simulink model "distributive4"  (R2022b)
settings: Solver=ode8  StartTime=0.0  StopTime=0.25  FixedStep=0.0001  RelTol=1e-3
values from neighbouring files (symbols this model uses):
  A = [a11,0;0,a22]    [distributive3.m]    (also in neurobserver4.m = [1 1;1 2])
  alpha = 0.9e-6    (= 9e-07)    [distributive3.m]
  amp = 80e-6    (= 8e-05)    [distributive3.m]
  angvel = (2*pi)*30    (= 188.495559215)    [distributive3.m]
  B = [b11,0;0,b22]    [distributive3.m]    (also in neurobserver4.m = 1000)
  beta = 0.008    [distributive3.m]
  C = [1,0]    [distributive3.m]
  C_bar = [1,0]    [distributive3.m]    (also in neurobserver4.m = [1,0;0,1])
  d_p = 1.6e-6    (= 1.6e-06)    [distributive3.m]
  fase = 2*pi/10    (= 0.628318530718)    [distributive3.m]
  G = S\C_bar'    [distributive3.m]    (also in neurobserver4.m)
  gamma = 0.008    [distributive3.m]
  Gamma = [0,-B;0 0]    [distributive3.m]    (also in neurobserver4.m = [ 0 , -B ; 0 , 0 ])
  h = legend('Closed-loop response map $(y_d,y)$')    [distributive3.m]    (also in neurobserver4.m = legend('$(y_r,y)$ for $x=7.5$, $f=1Hz$','$(y_r,y)$ for $x=15)
  h_i = 2e-6    (= 2e-06)    [distributive3.m]
  k1 = 7    [distributive3.m]    (also in neurobserver4.m)
  k2 = 7    [distributive3.m]    (also in neurobserver4.m)
  kappa1 = 4e3    (= 4000)    [distributive3.m]    (also in neurobserver4.m = 120)
  L = 20000    [distributive3.m]
  S = [s11,s12;s21,s22]    [distributive3.m]    (also in neurobserver4.m = [1/theta,B/theta^2;B/theta^2,(2*B^2)/theta^3])
  V = learning.V    [neurobserver4.m]
  W = learning.W    [neurobserver4.m]
  x1 = e(2)    [distributive3.m]
  x2 = e(5)    [distributive3.m]
  y_i = -3e-6    (= -3e-06)    [distributive3.m]
undefined symbols (not defined in the file or in its folder): freq, Gamma_c, Y
(part 2 of 3)

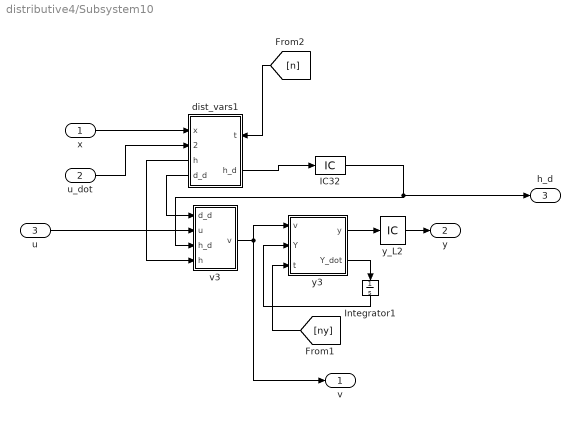
== system distributive4/Subsystem10 ==
  x : Inport
  u_dot : Inport  Port=2
  u : Inport  Port=3
  IC32 : InitialCondition  Value=h_i
  Integrator1 : Integrator
  dist_vars1 : Subsystem
      settings: PortSchema="{\"entries\":[{\"content\":{\"sides\":[{\"content\":{\"connectorIds\":[\"In1\",\"In2\",\"Out2\",\"Out3\"]},\"type\":\"ConnectorPlacement.EquallySpacedRectSide\",\"uuid\":\"c6804a03-85ed-4e19-a8b2-23b3b91cc999\"},{\"content\":{\"connectorIds\":[\"In3\",\"Out1\"],\"side\":\"RIGHT\"},\"type\":\"ConnectorPlacement.EquallySpacedRectSide\",\"uuid\":\"3893e005-dabd-44b9-aa2f-690b9b6a2b6d\"},{\"content\":{\"connectorIds\":[],\"side\":\"TOP\"},\"type\":\"ConnectorPlacement.EquallySpacedRectSide\",\"uuid\":\"9986ad97-c002-4a16-bb79-a95333cc5799\"}]},\"type\":\"ConnectorPlacement.EquallySpacedConnector\",\"uuid\":\"d796f436-4cc2-4114-998c-ef0d57f68d4d\"}],\"packageUris\":[\"http://schema.mathworks.com/mf0/Connector/R2020b\"],\"version\":\"1.0\"}"
  v3 : MATLAB Function  TreatAsAtomicUnit=on
  y3 : MATLAB Function  TreatAsAtomicUnit=on
  y_L2 : InitialCondition  Value=[y_i;0]
  v : Outport
  y : Outport  Port=2
  h_d : Outport  Port=3
  wires:
  dist_vars1/3(d_d) -> v3/1(d_d)
  v3/1(v) -> y3/1(v), v/1
  y3/2(Y_dot) -> Integrator1/1
  IC32/1 -> v3/3(h_d), h_d/1
  dist_vars1/2(h) -> v3/4(h)
  dist_vars1/1(h_d) -> IC32/1
  y3/1(y) -> y_L2/1
  [n] -> dist_vars1/3(t)
  Integrator1/1 -> y3/2(Y)
  [ny] -> y3/3(t)
  u_dot/1 -> dist_vars1/2(u_dot)
  x/1 -> dist_vars1/1(x)
  u/1 -> v3/2(u)
  y_L2/1 -> y/1

== system distributive4/Subsystem11 ==
  x : Inport
  y_ref : Inport  Port=2
  z_hat : Inport  Port=3
  d_d : Inport  Port=4
  Derivative32 : Derivative
  h_d_ref14 : MATLAB Function  TreatAsAtomicUnit=on
  u_ref13 : Integrator
  u_ref_dot14 : MATLAB Function  TreatAsAtomicUnit=on
  u_ref_dot : Outport
  u_ref : Outport  Port=2
  h_d_ref : Outport  Port=3
  wires:
  z_hat/1 -> h_d_ref14/4(z_hat), u_ref_dot14/2(z_hat)
  u_ref13/1 -> u_ref/1, h_d_ref14/1(u)
  Derivative32/1 -> h_d_ref14/3(y_ref_dot)
  x/1 -> u_ref_dot14/3(x)
  h_d_ref14/1(h_d_ref) -> u_ref_dot14/1(h_d_ref), h_d_ref/1
  u_ref_dot14/1(u_ref_dot) -> u_ref13/1, u_ref_dot/1
  d_d/1 -> h_d_ref14/5(d_d)
  y_ref/1 -> Derivative32/1, h_d_ref14/2(y_ref)

== system distributive4/Subsystem12 ==
  x : Inport
  y : Inport  Port=2
  u_dot : Inport  Port=3
  u : Inport  Port=4
  Integrator14 : Integrator  InitialCondition=[0;0]
  dist_vars15 : Subsystem
      settings: PortSchema="{\"entries\":[{\"content\":{\"sides\":[{\"content\":{\"connectorIds\":[\"In1\",\"In2\",\"Out1\",\"Out2\",\"Out3\"]},\"type\":\"ConnectorPlacement.EquallySpacedRectSide\",\"uuid\":\"c6804a03-85ed-4e19-a8b2-23b3b91cc999\"},{\"content\":{\"connectorIds\":[],\"side\":\"RIGHT\"},\"type\":\"ConnectorPlacement.EquallySpacedRectSide\",\"uuid\":\"3893e005-dabd-44b9-aa2f-690b9b6a2b6d\"},{\"content\":{\"connectorIds\":[],\"side\":\"TOP\"},\"type\":\"ConnectorPlacement.EquallySpacedRectSide\",\"uuid\":\"9986ad97-c002-4a16-bb79-a95333cc5799\"}]},\"type\":\"ConnectorPlacement.EquallySpacedConnector\",\"uuid\":\"d796f436-4cc2-4114-998c-ef0d57f68d4d\"}],\"packageUris\":[\"http://schema.mathworks.com/mf0/Connector/R2020b\"],\"version\":\"1.0\"}"
  observer5 : MATLAB Function  TreatAsAtomicUnit=on
  d_d : Outport
  z_hat : Outport  Port=2
  wires:
  observer5/1(z_hat_dot) -> Integrator14/1
  u/1 -> observer5/5(u)
  dist_vars15/3(h_d) -> observer5/4(h_d)
  dist_vars15/2(d_d) -> observer5/7(d_d), d_d/1
  dist_vars15/1(h_d_dot) -> observer5/6(h_d_dot)
  Integrator14/1 -> observer5/1(z_hat), z_hat/1
  u_dot/1 -> dist_vars15/1(u_dot)
  y/1 -> observer5/2(y)
  x/1 -> dist_vars15/2(x), observer5/3(x)

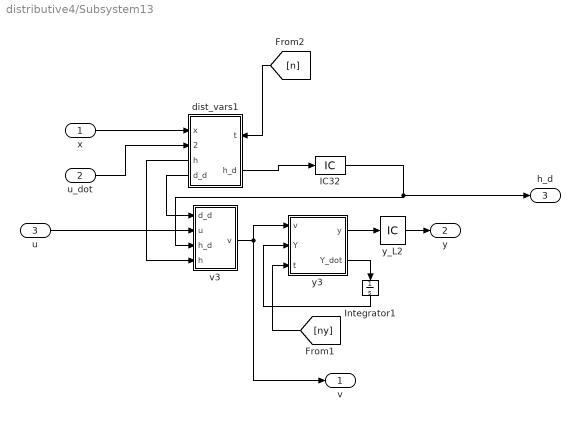
== system distributive4/Subsystem13 ==
  x : Inport
  u_dot : Inport  Port=2
  u : Inport  Port=3
  IC32 : InitialCondition  Value=h_i
  Integrator1 : Integrator
  dist_vars1 : Subsystem
      settings: PortSchema="{\"entries\":[{\"content\":{\"sides\":[{\"content\":{\"connectorIds\":[\"In1\",\"In2\",\"Out2\",\"Out3\"]},\"type\":\"ConnectorPlacement.EquallySpacedRectSide\",\"uuid\":\"c6804a03-85ed-4e19-a8b2-23b3b91cc999\"},{\"content\":{\"connectorIds\":[\"In3\",\"Out1\"],\"side\":\"RIGHT\"},\"type\":\"ConnectorPlacement.EquallySpacedRectSide\",\"uuid\":\"3893e005-dabd-44b9-aa2f-690b9b6a2b6d\"},{\"content\":{\"connectorIds\":[],\"side\":\"TOP\"},\"type\":\"ConnectorPlacement.EquallySpacedRectSide\",\"uuid\":\"9986ad97-c002-4a16-bb79-a95333cc5799\"}]},\"type\":\"ConnectorPlacement.EquallySpacedConnector\",\"uuid\":\"d796f436-4cc2-4114-998c-ef0d57f68d4d\"}],\"packageUris\":[\"http://schema.mathworks.com/mf0/Connector/R2020b\"],\"version\":\"1.0\"}"
  v3 : MATLAB Function  TreatAsAtomicUnit=on
  y3 : MATLAB Function  TreatAsAtomicUnit=on
  y_L2 : InitialCondition  Value=[y_i;0]
  v : Outport
  y : Outport  Port=2
  h_d : Outport  Port=3
  wires:
  dist_vars1/3(d_d) -> v3/1(d_d)
  v3/1(v) -> y3/1(v), v/1
  y3/2(Y_dot) -> Integrator1/1
  IC32/1 -> v3/3(h_d), h_d/1
  dist_vars1/2(h) -> v3/4(h)
  dist_vars1/1(h_d) -> IC32/1
  y3/1(y) -> y_L2/1
  [n] -> dist_vars1/3(t)
  Integrator1/1 -> y3/2(Y)
  [ny] -> y3/3(t)
  u_dot/1 -> dist_vars1/2(u_dot)
  x/1 -> dist_vars1/1(x)
  u/1 -> v3/2(u)
  y_L2/1 -> y/1

== system distributive4/Subsystem14 ==
  x : Inport
  y_ref : Inport  Port=2
  z_hat : Inport  Port=3
  d_d : Inport  Port=4
  Derivative32 : Derivative
  h_d_ref14 : MATLAB Function  TreatAsAtomicUnit=on
  u_ref13 : Integrator
  u_ref_dot14 : MATLAB Function  TreatAsAtomicUnit=on
  u_ref_dot : Outport
  u_ref : Outport  Port=2
  h_d_ref : Outport  Port=3
  wires:
  z_hat/1 -> h_d_ref14/4(z_hat), u_ref_dot14/2(z_hat)
  u_ref13/1 -> u_ref/1, h_d_ref14/1(u)
  Derivative32/1 -> h_d_ref14/3(y_ref_dot)
  x/1 -> u_ref_dot14/3(x)
  h_d_ref14/1(h_d_ref) -> u_ref_dot14/1(h_d_ref), h_d_ref/1
  u_ref_dot14/1(u_ref_dot) -> u_ref13/1, u_ref_dot/1
  d_d/1 -> h_d_ref14/5(d_d)
  y_ref/1 -> Derivative32/1, h_d_ref14/2(y_ref)

== system distributive4/Subsystem15 ==
  x : Inport
  y : Inport  Port=2
  u_dot : Inport  Port=3
  u : Inport  Port=4
  Integrator14 : Integrator  InitialCondition=[0;0]
  dist_vars15 : Subsystem
      settings: PortSchema="{\"entries\":[{\"content\":{\"sides\":[{\"content\":{\"connectorIds\":[\"In1\",\"In2\",\"Out1\",\"Out2\",\"Out3\"]},\"type\":\"ConnectorPlacement.EquallySpacedRectSide\",\"uuid\":\"c6804a03-85ed-4e19-a8b2-23b3b91cc999\"},{\"content\":{\"connectorIds\":[],\"side\":\"RIGHT\"},\"type\":\"ConnectorPlacement.EquallySpacedRectSide\",\"uuid\":\"3893e005-dabd-44b9-aa2f-690b9b6a2b6d\"},{\"content\":{\"connectorIds\":[],\"side\":\"TOP\"},\"type\":\"ConnectorPlacement.EquallySpacedRectSide\",\"uuid\":\"9986ad97-c002-4a16-bb79-a95333cc5799\"}]},\"type\":\"ConnectorPlacement.EquallySpacedConnector\",\"uuid\":\"d796f436-4cc2-4114-998c-ef0d57f68d4d\"}],\"packageUris\":[\"http://schema.mathworks.com/mf0/Connector/R2020b\"],\"version\":\"1.0\"}"
  observer5 : MATLAB Function  TreatAsAtomicUnit=on
  d_d : Outport
  z_hat : Outport  Port=2
  wires:
  observer5/1(z_hat_dot) -> Integrator14/1
  u/1 -> observer5/5(u)
  dist_vars15/3(h_d) -> observer5/4(h_d)
  dist_vars15/2(d_d) -> observer5/7(d_d), d_d/1
  dist_vars15/1(h_d_dot) -> observer5/6(h_d_dot)
  Integrator14/1 -> observer5/1(z_hat), z_hat/1
  u_dot/1 -> dist_vars15/1(u_dot)
  y/1 -> observer5/2(y)
  x/1 -> dist_vars15/2(x), observer5/3(x)

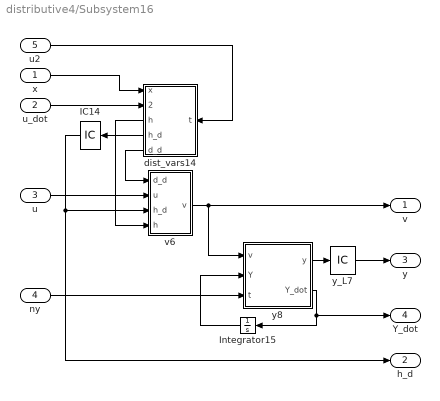
== system distributive4/Subsystem16 ==
  x : Inport
  u_dot : Inport  Port=2
  u : Inport  Port=3
  ny : Inport  Port=4
  u2 : Inport  Port=5
  IC14 : InitialCondition  Value=h_i
  Integrator15 : Integrator
  dist_vars14 : Subsystem
      settings: PortSchema="{\"entries\":[{\"content\":{\"sides\":[{\"content\":{\"connectorIds\":[\"In1\",\"In2\",\"Out1\",\"Out2\",\"Out3\"]},\"type\":\"ConnectorPlacement.EquallySpacedRectSide\",\"uuid\":\"c6804a03-85ed-4e19-a8b2-23b3b91cc999\"},{\"content\":{\"connectorIds\":[\"In3\"],\"side\":\"RIGHT\"},\"type\":\"ConnectorPlacement.EquallySpacedRectSide\",\"uuid\":\"3893e005-dabd-44b9-aa2f-690b9b6a2b6d\"},{\"content\":{\"connectorIds\":[],\"side\":\"TOP\"},\"type\":\"ConnectorPlacement.EquallySpacedRectSide\",\"uuid\":\"9986ad97-c002-4a16-bb79-a95333cc5799\"}]},\"type\":\"ConnectorPlacement.EquallySpacedConnector\",\"uuid\":\"d796f436-4cc2-4114-998c-ef0d57f68d4d\"}],\"packageUris\":[\"http://schema.mathworks.com/mf0/Connector/R2020b\"],\"version\":\"1.0\"}"
  v6 : MATLAB Function  TreatAsAtomicUnit=on
  y8 : MATLAB Function  TreatAsAtomicUnit=on
  y_L7 : InitialCondition  Value=[y_i;0]
  v : Outport
  h_d : Outport  Port=2
  y : Outport  Port=3
  Y_dot : Outport  Port=4
  wires:
  u2/1 -> dist_vars14/3(t)
  y_L7/1 -> y/1
  Integrator15/1 -> y8/2(Y)
  dist_vars14/3(d_d) -> v6/1(d_d)
  y8/2(Y_dot) -> Integrator15/1, Y_dot/1
  v6/1(v) -> v/1, y8/1(v)
  dist_vars14/1(h) -> v6/4(h)
  y8/1(y) -> y_L7/1
  dist_vars14/2(h_d) -> IC14/1
  x/1 -> dist_vars14/1(x)
  ny/1 -> y8/3(t)
  u/1 -> v6/2(u)
  IC14/1 -> v6/3(h_d), h_d/1
  u_dot/1 -> dist_vars14/2(u_dot)

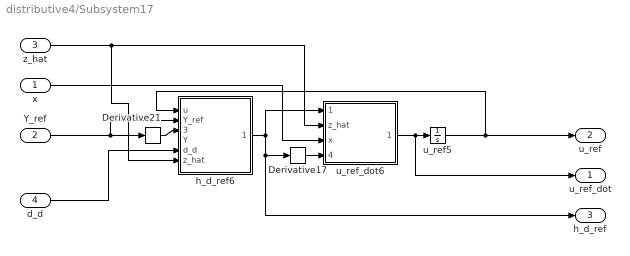
== system distributive4/Subsystem17 ==
  x : Inport
  Y_ref : Inport  Port=2
  z_hat : Inport  Port=3
  d_d : Inport  Port=4
  Derivative17 : Derivative
  Derivative21 : Derivative
  h_d_ref6 : MATLAB Function  TreatAsAtomicUnit=on
  u_ref5 : Integrator
  u_ref_dot6 : MATLAB Function  TreatAsAtomicUnit=on
  u_ref_dot : Outport
  u_ref : Outport  Port=2
  h_d_ref : Outport  Port=3
  wires:
  Derivative21/1 -> h_d_ref6/3(Y_ref_dot)
  Y_ref/1 -> h_d_ref6/2(Y_ref), Derivative21/1
  u_ref5/1 -> h_d_ref6/1(u), u_ref/1
  Derivative17/1 -> u_ref_dot6/4(h_d_dot)
  h_d_ref6/1(h_d_ref) -> u_ref_dot6/1(h_d_ref), h_d_ref/1, Derivative17/1
  u_ref_dot6/1(u_ref_dot) -> u_ref_dot/1, u_ref5/1
  x/1 -> u_ref_dot6/3(x)
  d_d/1 -> h_d_ref6/5(d_d)
  z_hat/1 -> h_d_ref6/6(z_hat), u_ref_dot6/2(z_hat)

== system distributive4/Subsystem2 ==
  y_ref : Inport
  x : Inport  Port=2
  u : Inport  Port=3
  Derivative5 : Derivative
  Subsystem4 : Subsystem
  inv D3 : MATLAB Function  TreatAsAtomicUnit=on
  inv v3 : MATLAB Function  TreatAsAtomicUnit=on
  y_d_hat : Outport
  u_dot : Outport  Port=2
  u_ref : Outport  Port=3
  wires:
  y_ref/1 -> inv D3/1(y_ref)
  inv v3/1(u_ref) -> u_ref/1
  Subsystem4/4(u_dot) -> u_dot/1
  inv D3/2(Y) -> Derivative5/1
  Derivative5/1 -> inv D3/2(Y_dot)
  Subsystem4/1(d_d_hat) -> inv v3/3(d_d)
  Subsystem4/3(h_d_hat) -> inv v3/2(h_d)
  inv D3/1(v_ref) -> inv v3/1(v)
  Subsystem4/2(y_d_hat) -> y_d_hat/1
  x/1 -> Subsystem4/1(x)
  u/1 -> Subsystem4/2(u)

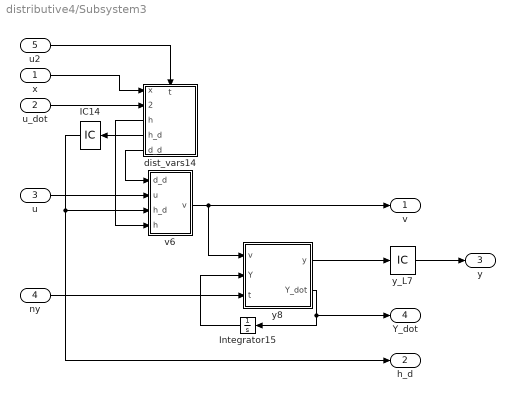
== system distributive4/Subsystem3 ==
  x : Inport
  u_dot : Inport  Port=2
  u : Inport  Port=3
  ny : Inport  Port=4
  u2 : Inport  Port=5
  IC14 : InitialCondition  Value=h_i
  Integrator15 : Integrator
  dist_vars14 : Subsystem
      settings: PortSchema="{\"entries\":[{\"content\":{\"sides\":[{\"content\":{\"connectorIds\":[\"In1\",\"In2\",\"Out1\",\"Out2\",\"Out3\"]},\"type\":\"ConnectorPlacement.EquallySpacedRectSide\",\"uuid\":\"c6804a03-85ed-4e19-a8b2-23b3b91cc999\"},{\"content\":{\"connectorIds\":[],\"side\":\"RIGHT\"},\"type\":\"ConnectorPlacement.EquallySpacedRectSide\",\"uuid\":\"3893e005-dabd-44b9-aa2f-690b9b6a2b6d\"},{\"content\":{\"connectorIds\":[\"In3\"],\"side\":\"TOP\"},\"type\":\"ConnectorPlacement.EquallySpacedRectSide\",\"uuid\":\"9986ad97-c002-4a16-bb79-a95333cc5799\"}]},\"type\":\"ConnectorPlacement.EquallySpacedConnector\",\"uuid\":\"d796f436-4cc2-4114-998c-ef0d57f68d4d\"}],\"packageUris\":[\"http://schema.mathworks.com/mf0/Connector/R2020b\"],\"version\":\"1.0\"}"
  v6 : MATLAB Function  TreatAsAtomicUnit=on
  y8 : MATLAB Function  TreatAsAtomicUnit=on
  y_L7 : InitialCondition  Value=[y_i;0]
  v : Outport
  h_d : Outport  Port=2
  y : Outport  Port=3
  Y_dot : Outport  Port=4
  wires:
  u2/1 -> dist_vars14/3(t)
  y_L7/1 -> y/1
  Integrator15/1 -> y8/2(Y)
  dist_vars14/3(d_d) -> v6/1(d_d)
  y8/2(Y_dot) -> Integrator15/1, Y_dot/1
  v6/1(v) -> v/1, y8/1(v)
  dist_vars14/1(h) -> v6/4(h)
  y8/1(y) -> y_L7/1
  dist_vars14/2(h_d) -> IC14/1
  x/1 -> dist_vars14/1(x)
  ny/1 -> y8/3(t)
  u/1 -> v6/2(u)
  IC14/1 -> v6/3(h_d), h_d/1
  u_dot/1 -> dist_vars14/2(u_dot)

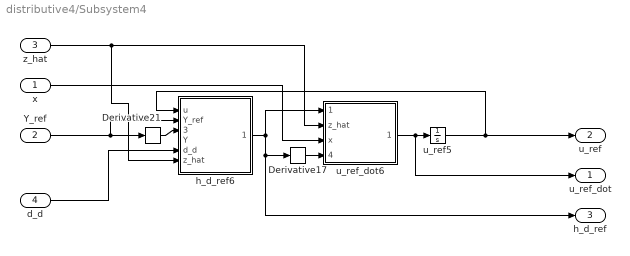
== system distributive4/Subsystem4 ==
  x : Inport
  Y_ref : Inport  Port=2
  z_hat : Inport  Port=3
  d_d : Inport  Port=4
  Derivative17 : Derivative
  Derivative21 : Derivative
  h_d_ref6 : MATLAB Function  TreatAsAtomicUnit=on
  u_ref5 : Integrator
  u_ref_dot6 : MATLAB Function  TreatAsAtomicUnit=on
  u_ref_dot : Outport
  u_ref : Outport  Port=2
  h_d_ref : Outport  Port=3
  wires:
  Derivative21/1 -> h_d_ref6/3(Y_ref_dot)
  Y_ref/1 -> h_d_ref6/2(Y_ref), Derivative21/1
  u_ref5/1 -> h_d_ref6/1(u), u_ref/1
  Derivative17/1 -> u_ref_dot6/4(h_d_dot)
  h_d_ref6/1(h_d_ref) -> u_ref_dot6/1(h_d_ref), h_d_ref/1, Derivative17/1
  u_ref_dot6/1(u_ref_dot) -> u_ref_dot/1, u_ref5/1
  x/1 -> u_ref_dot6/3(x)
  d_d/1 -> h_d_ref6/5(d_d)
  z_hat/1 -> h_d_ref6/6(z_hat), u_ref_dot6/2(z_hat)

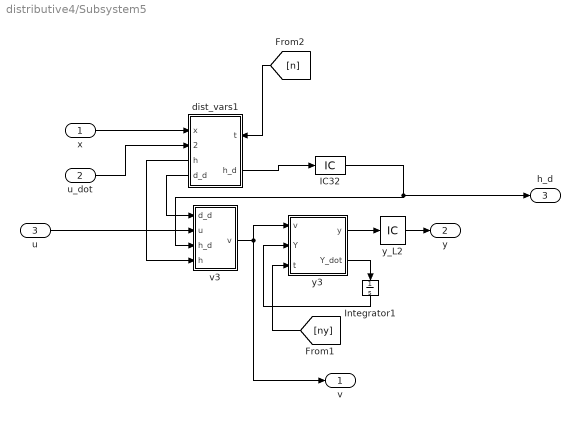
== system distributive4/Subsystem5 ==
  x : Inport
  u_dot : Inport  Port=2
  u : Inport  Port=3
  IC32 : InitialCondition  Value=h_i
  Integrator1 : Integrator
  dist_vars1 : Subsystem
      settings: PortSchema="{\"entries\":[{\"content\":{\"sides\":[{\"content\":{\"connectorIds\":[\"In1\",\"In2\",\"Out2\",\"Out3\"]},\"type\":\"ConnectorPlacement.EquallySpacedRectSide\",\"uuid\":\"c6804a03-85ed-4e19-a8b2-23b3b91cc999\"},{\"content\":{\"connectorIds\":[\"In3\",\"Out1\"],\"side\":\"RIGHT\"},\"type\":\"ConnectorPlacement.EquallySpacedRectSide\",\"uuid\":\"3893e005-dabd-44b9-aa2f-690b9b6a2b6d\"},{\"content\":{\"connectorIds\":[],\"side\":\"TOP\"},\"type\":\"ConnectorPlacement.EquallySpacedRectSide\",\"uuid\":\"9986ad97-c002-4a16-bb79-a95333cc5799\"}]},\"type\":\"ConnectorPlacement.EquallySpacedConnector\",\"uuid\":\"d796f436-4cc2-4114-998c-ef0d57f68d4d\"}],\"packageUris\":[\"http://schema.mathworks.com/mf0/Connector/R2020b\"],\"version\":\"1.0\"}"
  v3 : MATLAB Function  TreatAsAtomicUnit=on
  y3 : MATLAB Function  TreatAsAtomicUnit=on
  y_L2 : InitialCondition  Value=[y_i;0]
  v : Outport
  y : Outport  Port=2
  h_d : Outport  Port=3
  wires:
  dist_vars1/3(d_d) -> v3/1(d_d)
  v3/1(v) -> y3/1(v), v/1
  y3/2(Y_dot) -> Integrator1/1
  IC32/1 -> v3/3(h_d), h_d/1
  dist_vars1/2(h) -> v3/4(h)
  dist_vars1/1(h_d) -> IC32/1
  y3/1(y) -> y_L2/1
  [n] -> dist_vars1/3(t)
  Integrator1/1 -> y3/2(Y)
  [ny] -> y3/3(t)
  u_dot/1 -> dist_vars1/2(u_dot)
  x/1 -> dist_vars1/1(x)
  u/1 -> v3/2(u)
  y_L2/1 -> y/1

== system distributive4/Subsystem6 ==
  x : Inport
  y_ref : Inport  Port=2
  z_hat : Inport  Port=3
  d_d : Inport  Port=4
  Derivative32 : Derivative
  h_d_ref14 : MATLAB Function  TreatAsAtomicUnit=on
  u_ref13 : Integrator
  u_ref_dot14 : MATLAB Function  TreatAsAtomicUnit=on
  u_ref_dot : Outport
  u_ref : Outport  Port=2
  h_d_ref : Outport  Port=3
  wires:
  z_hat/1 -> h_d_ref14/4(z_hat), u_ref_dot14/2(z_hat)
  u_ref13/1 -> u_ref/1, h_d_ref14/1(u)
  Derivative32/1 -> h_d_ref14/3(y_ref_dot)
  x/1 -> u_ref_dot14/3(x)
  h_d_ref14/1(h_d_ref) -> u_ref_dot14/1(h_d_ref), h_d_ref/1
  u_ref_dot14/1(u_ref_dot) -> u_ref13/1, u_ref_dot/1
  d_d/1 -> h_d_ref14/5(d_d)
  y_ref/1 -> Derivative32/1, h_d_ref14/2(y_ref)

== system distributive4/Subsystem7 ==
  x : Inport
  y : Inport  Port=2
  u_dot : Inport  Port=3
  u : Inport  Port=4
  Integrator14 : Integrator  InitialCondition=[0;0]
  dist_vars15 : Subsystem
      settings: PortSchema="{\"entries\":[{\"content\":{\"sides\":[{\"content\":{\"connectorIds\":[\"In1\",\"In2\",\"Out1\",\"Out2\",\"Out3\"]},\"type\":\"ConnectorPlacement.EquallySpacedRectSide\",\"uuid\":\"c6804a03-85ed-4e19-a8b2-23b3b91cc999\"},{\"content\":{\"connectorIds\":[],\"side\":\"RIGHT\"},\"type\":\"ConnectorPlacement.EquallySpacedRectSide\",\"uuid\":\"3893e005-dabd-44b9-aa2f-690b9b6a2b6d\"},{\"content\":{\"connectorIds\":[],\"side\":\"TOP\"},\"type\":\"ConnectorPlacement.EquallySpacedRectSide\",\"uuid\":\"9986ad97-c002-4a16-bb79-a95333cc5799\"}]},\"type\":\"ConnectorPlacement.EquallySpacedConnector\",\"uuid\":\"d796f436-4cc2-4114-998c-ef0d57f68d4d\"}],\"packageUris\":[\"http://schema.mathworks.com/mf0/Connector/R2020b\"],\"version\":\"1.0\"}"
  observer5 : MATLAB Function  TreatAsAtomicUnit=on
  d_d : Outport
  z_hat : Outport  Port=2
  wires:
  observer5/1(z_hat_dot) -> Integrator14/1
  u/1 -> observer5/5(u)
  dist_vars15/3(h_d) -> observer5/4(h_d)
  dist_vars15/2(d_d) -> observer5/7(d_d), d_d/1
  dist_vars15/1(h_d_dot) -> observer5/6(h_d_dot)
  Integrator14/1 -> observer5/1(z_hat), z_hat/1
  u_dot/1 -> dist_vars15/1(u_dot)
  y/1 -> observer5/2(y)
  x/1 -> dist_vars15/2(x), observer5/3(x)

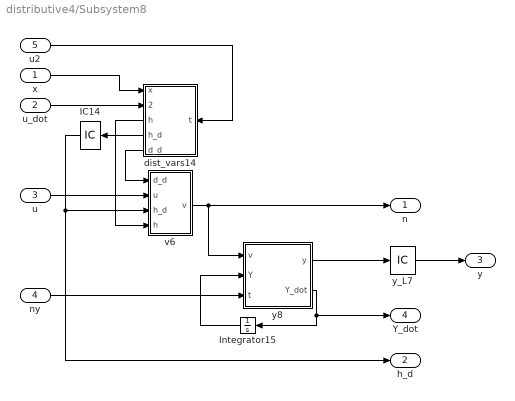
== system distributive4/Subsystem8 ==
  x : Inport
  u_dot : Inport  Port=2
  u : Inport  Port=3
  ny : Inport  Port=4
  u2 : Inport  Port=5
  IC14 : InitialCondition  Value=h_i
  Integrator15 : Integrator
  dist_vars14 : Subsystem
      settings: PortSchema="{\"entries\":[{\"content\":{\"sides\":[{\"content\":{\"connectorIds\":[\"In1\",\"In2\",\"Out1\",\"Out2\",\"Out3\"]},\"type\":\"ConnectorPlacement.EquallySpacedRectSide\",\"uuid\":\"c6804a03-85ed-4e19-a8b2-23b3b91cc999\"},{\"content\":{\"connectorIds\":[\"In3\"],\"side\":\"RIGHT\"},\"type\":\"ConnectorPlacement.EquallySpacedRectSide\",\"uuid\":\"3893e005-dabd-44b9-aa2f-690b9b6a2b6d\"},{\"content\":{\"connectorIds\":[],\"side\":\"TOP\"},\"type\":\"ConnectorPlacement.EquallySpacedRectSide\",\"uuid\":\"9986ad97-c002-4a16-bb79-a95333cc5799\"}]},\"type\":\"ConnectorPlacement.EquallySpacedConnector\",\"uuid\":\"d796f436-4cc2-4114-998c-ef0d57f68d4d\"}],\"packageUris\":[\"http://schema.mathworks.com/mf0/Connector/R2020b\"],\"version\":\"1.0\"}"
  v6 : MATLAB Function  TreatAsAtomicUnit=on
  y8 : MATLAB Function  TreatAsAtomicUnit=on
  y_L7 : InitialCondition  Value=[y_i;0]
  n : Outport
  h_d : Outport  Port=2
  y : Outport  Port=3
  Y_dot : Outport  Port=4
  wires:
  u2/1 -> dist_vars14/3(t)
  y_L7/1 -> y/1
  Integrator15/1 -> y8/2(Y)
  dist_vars14/3(d_d) -> v6/1(d_d)
  y8/2(Y_dot) -> Integrator15/1, Y_dot/1
  v6/1(v) -> n/1, y8/1(v)
  dist_vars14/1(h) -> v6/4(h)
  y8/1(y) -> y_L7/1
  dist_vars14/2(h_d) -> IC14/1
  x/1 -> dist_vars14/1(x)
  ny/1 -> y8/3(t)
  u/1 -> v6/2(u)
  IC14/1 -> v6/3(h_d), h_d/1
  u_dot/1 -> dist_vars14/2(u_dot)

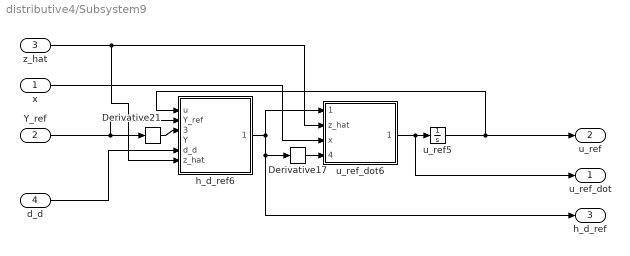
== system distributive4/Subsystem9 ==
  x : Inport
  Y_ref : Inport  Port=2
  z_hat : Inport  Port=3
  d_d : Inport  Port=4
  Derivative17 : Derivative
  Derivative21 : Derivative
  h_d_ref6 : MATLAB Function  TreatAsAtomicUnit=on
  u_ref5 : Integrator
  u_ref_dot6 : MATLAB Function  TreatAsAtomicUnit=on
  u_ref_dot : Outport
  u_ref : Outport  Port=2
  h_d_ref : Outport  Port=3
  wires:
  Derivative21/1 -> h_d_ref6/3(Y_ref_dot)
  Y_ref/1 -> h_d_ref6/2(Y_ref), Derivative21/1
  u_ref5/1 -> h_d_ref6/1(u), u_ref/1
  Derivative17/1 -> u_ref_dot6/4(h_d_dot)
  h_d_ref6/1(h_d_ref) -> u_ref_dot6/1(h_d_ref), h_d_ref/1, Derivative17/1
  u_ref_dot6/1(u_ref_dot) -> u_ref_dot/1, u_ref5/1
  x/1 -> u_ref_dot6/3(x)
  d_d/1 -> h_d_ref6/5(d_d)
  z_hat/1 -> h_d_ref6/6(z_hat), u_ref_dot6/2(z_hat)

== system distributive4/dist_vars11 ==
  note: h_d1
  x : Inport
  u : Inport  Port=2
  Derivative1 : Derivative
  Integrator1 : Integrator
  MATLAB Function : MATLAB Function  TreatAsAtomicUnit=on
  MATLAB Function5 : MATLAB Function  TreatAsAtomicUnit=on
  h_d_dot : Outport
  h_d : Outport  Port=2
  d_d : Outport  Port=3
  wires:
  Integrator1/1 -> MATLAB Function5/2(h)
  MATLAB Function5/1(h_dot) -> Integrator1/1
  x/1 -> MATLAB Function5/3(x), MATLAB Function/1(x)
  MATLAB Function/1(d_d) -> d_d/1
  MATLAB Function5/2(h_d) -> h_d/1
  u/1 -> Derivative1/1
  MATLAB Function5/3(h_d_dot) -> h_d_dot/1
  Derivative1/1 -> MATLAB Function5/1(u_dot)

== system distributive4/dist_vars22 ==
  x : Inport
  u_dot : Inport  Port=2
  Integrator1 : Integrator
  MATLAB Function : MATLAB Function  TreatAsAtomicUnit=on
  MATLAB Function5 : MATLAB Function  TreatAsAtomicUnit=on
  d_d : Outport
  h_d_dot : Outport  Port=2
  h_d : Outport  Port=3
  wires:
  Integrator1/1 -> MATLAB Function5/2(h)
  MATLAB Function5/1(h_dot) -> Integrator1/1
  u_dot/1 -> MATLAB Function5/1(u_dot)
  MATLAB Function/1(d_d) -> d_d/1
  MATLAB Function5/2(h_d) -> h_d/1
  x/1 -> MATLAB Function5/3(x), MATLAB Function/1(x)
  MATLAB Function5/3(h_d_dot) -> h_d_dot/1

== system distributive4/dist_vars23 ==
  x : Inport
  u_dot : Inport  Port=2
  Integrator1 : Integrator
  MATLAB Function : MATLAB Function  TreatAsAtomicUnit=on
  MATLAB Function5 : MATLAB Function  TreatAsAtomicUnit=on
  d_d : Outport
  h_d_dot : Outport  Port=2
  h_d : Outport  Port=3
  wires:
  Integrator1/1 -> MATLAB Function5/2(h)
  MATLAB Function5/1(h_dot) -> Integrator1/1
  u_dot/1 -> MATLAB Function5/1(u_dot)
  MATLAB Function/1(d_d) -> d_d/1
  MATLAB Function5/2(h_d) -> h_d/1
  x/1 -> MATLAB Function5/3(x), MATLAB Function/1(x)
  MATLAB Function5/3(h_d_dot) -> h_d_dot/1

== system distributive4/dist_vars24 ==
  x : Inport
  u_dot : Inport  Port=2
  Clock : Clock
  Integrator1 : Integrator
  MATLAB Function : MATLAB Function  TreatAsAtomicUnit=on
  MATLAB Function5 : MATLAB Function  TreatAsAtomicUnit=on
  Sum : Sum  Inputs=|++
  disturbances : MATLAB Function  TreatAsAtomicUnit=on
  d_d : Outport
  h_d : Outport  Port=2
  h_d_dot : Outport  Port=3
  wires:
  Integrator1/1 -> MATLAB Function5/2(h)
  x/1 -> MATLAB Function5/3(x), MATLAB Function/1(x)
  MATLAB Function/1(d_d) -> d_d/1
  MATLAB Function5/2(h_d) -> h_d/1
  u_dot/1 -> MATLAB Function5/1(u_dot)
  MATLAB Function5/3(h_d_dot) -> h_d_dot/1
  Clock/1 -> disturbances/1(t)
  disturbances/1(delta) -> Sum/1
  MATLAB Function5/1(h_dot) -> Sum/2
  Sum/1 -> Integrator1/1

== system distributive4/dist_vars25 ==
  x : Inport
  u_dot : Inport  Port=2
  Clock : Clock
  Integrator1 : Integrator
  MATLAB Function : MATLAB Function  TreatAsAtomicUnit=on
  MATLAB Function5 : MATLAB Function  TreatAsAtomicUnit=on
  Sum : Sum  Inputs=|++
  disturbances : MATLAB Function  TreatAsAtomicUnit=on
  d_d : Outport
  h_d : Outport  Port=2
  h_d_dot : Outport  Port=3
  wires:
  Integrator1/1 -> MATLAB Function5/2(h)
  x/1 -> MATLAB Function5/3(x), MATLAB Function/1(x)
  MATLAB Function/1(d_d) -> d_d/1
  MATLAB Function5/2(h_d) -> h_d/1
  u_dot/1 -> MATLAB Function5/1(u_dot)
  MATLAB Function5/3(h_d_dot) -> h_d_dot/1
  MATLAB Function5/1(h_dot) -> Sum/2
  Sum/1 -> Integrator1/1
  disturbances/1(delta) -> Sum/1
  Clock/1 -> disturbances/1(t)

== system distributive4/dist_vars3 ==
  note: h_d1
  x : Inport
  u_dot : Inport  Port=2
  Integrator1 : Integrator
  MATLAB Function : MATLAB Function  TreatAsAtomicUnit=on
  MATLAB Function5 : MATLAB Function  TreatAsAtomicUnit=on
  d_d : Outport
  h_d : Outport  Port=2
  h_d_dot : Outport  Port=3
  wires:
  Integrator1/1 -> MATLAB Function5/2(h)
  MATLAB Function5/1(h_dot) -> Integrator1/1
  x/1 -> MATLAB Function5/3(x), MATLAB Function/1(x)
  MATLAB Function/1(d_d) -> d_d/1
  MATLAB Function5/2(h_d) -> h_d/1
  u_dot/1 -> MATLAB Function5/1(u_dot)
  MATLAB Function5/3(h_d_dot) -> h_d_dot/1

== system distributive4/dist_vars36 ==
  x : Inport
  u_dot : Inport  Port=2
  Integrator1 : Integrator
  MATLAB Function : MATLAB Function  TreatAsAtomicUnit=on
  MATLAB Function5 : MATLAB Function  TreatAsAtomicUnit=on
  h_d_dot : Outport
  h_d : Outport  Port=2
  d_d : Outport  Port=3
  wires:
  Integrator1/1 -> MATLAB Function5/2(h)
  MATLAB Function5/1(h_dot) -> Integrator1/1
  u_dot/1 -> MATLAB Function5/1(u_dot)
  MATLAB Function/1(d_d) -> d_d/1
  MATLAB Function5/2(h_d) -> h_d/1
  x/1 -> MATLAB Function5/3(x), MATLAB Function/1(x)
  MATLAB Function5/3(h_d_dot) -> h_d_dot/1

== system distributive4/dist_vars37 ==
  x : Inport
  u_dot : Inport  Port=2
  Integrator1 : Integrator
  MATLAB Function : MATLAB Function  TreatAsAtomicUnit=on
  MATLAB Function5 : MATLAB Function  TreatAsAtomicUnit=on
  h_d_dot : Outport
  d_d : Outport  Port=2
  h_d : Outport  Port=3
  h : Outport  Port=4
  wires:
  Integrator1/1 -> h/1, MATLAB Function5/2(h)
  MATLAB Function5/1(h_dot) -> Integrator1/1
  x/1 -> MATLAB Function5/3(x), MATLAB Function/1(x)
  MATLAB Function/1(d_d) -> d_d/1
  MATLAB Function5/2(h_d) -> h_d/1
  u_dot/1 -> MATLAB Function5/1(u_dot)
  MATLAB Function5/3(h_d_dot) -> h_d_dot/1

== system distributive4/dist_vars39 ==
  x : Inport
  u_dot : Inport  Port=2
  t : Inport  Port=3
  Integrator1 : Integrator
  Integrator2 : Integrator
  MATLAB Function : MATLAB Function  TreatAsAtomicUnit=on
  MATLAB Function5 : MATLAB Function  TreatAsAtomicUnit=on
  h_d_dot : Outport
  d_d : Outport  Port=2
  h_d : Outport  Port=3
  wires:
  MATLAB Function5/2(h_d_dot) -> Integrator1/1, h_d_dot/1
  x/1 -> MATLAB Function5/3(x), MATLAB Function/1(x)
  MATLAB Function/1(d_d) -> d_d/1
  u_dot/1 -> MATLAB Function5/1(u_dot)
  Integrator1/1 -> h_d/1
  MATLAB Function5/1(h_dot) -> Integrator2/1
  Integrator2/1 -> MATLAB Function5/2(h)
  t/1 -> MATLAB Function5/4(t)

== system distributive4/dist_vars4 ==
  x : Inport
  IC : InitialCondition  Value=0.01
  MATLAB Function : MATLAB Function  TreatAsAtomicUnit=on
  Switch : Switch  Criteria=u2 > Threshold  SaturateOnIntegerOverflow=off  InputSameDT=off
  d_d : Outport
  wires:
  MATLAB Function/1(d_d) -> Switch/3, Switch/2, Switch/1
  Switch/1 -> IC/1
  x/1 -> MATLAB Function/1(x)
  IC/1 -> d_d/1

== system distributive4/dist_vars40 ==
  u_dot : Inport
  x : Inport  Port=2
  Integrator2 : Integrator
  Integrator3 : Integrator
  MATLAB Function : MATLAB Function  TreatAsAtomicUnit=on
  MATLAB Function1 : MATLAB Function  TreatAsAtomicUnit=on
  h_d : Outport
  h_d_dot : Outport  Port=2
  d_d : Outport  Port=3
  wires:
  MATLAB Function/1(d_d) -> d_d/1
  MATLAB Function1/1(h_dot) -> Integrator3/1
  u_dot/1 -> MATLAB Function1/1(u_dot)
  MATLAB Function1/2(h_d_dot) -> h_d_dot/1, Integrator2/1
  x/1 -> MATLAB Function1/3(x), MATLAB Function/1(x)
  Integrator3/1 -> MATLAB Function1/2(h)
  Integrator2/1 -> h_d/1

== system distributive4/dist_vars6 ==
  note: h_d1
  x : Inport
  u_dot : Inport  Port=2
  Integrator1 : Integrator
  MATLAB Function : MATLAB Function  TreatAsAtomicUnit=on
  MATLAB Function5 : MATLAB Function  TreatAsAtomicUnit=on
  d_d : Outport
  h_d : Outport  Port=2
  h_d_dot : Outport  Port=3
  wires:
  Integrator1/1 -> MATLAB Function5/2(h)
  MATLAB Function5/1(h_dot) -> Integrator1/1
  x/1 -> MATLAB Function5/3(x), MATLAB Function/1(x)
  MATLAB Function/1(d_d) -> d_d/1
  MATLAB Function5/2(h_d) -> h_d/1
  u_dot/1 -> MATLAB Function5/1(u_dot)
  MATLAB Function5/3(h_d_dot) -> h_d_dot/1

== system distributive4/measurements1 ==
  u : Inport
  u_dot : Inport  Port=2
  Integrator1 : Integrator
  MATLAB Function1 : MATLAB Function  TreatAsAtomicUnit=on
  MATLAB Function5 : MATLAB Function  TreatAsAtomicUnit=on
  y_L : Outport
  h : Outport  Port=2
  wires:
  Integrator1/1 -> h/1, MATLAB Function1/1(h), MATLAB Function5/2(h)
  MATLAB Function5/1(h_dot) -> Integrator1/1
  u/1 -> MATLAB Function1/2(u)
  MATLAB Function1/1(y_L) -> y_L/1
  u_dot/1 -> MATLAB Function5/1(u_dot)

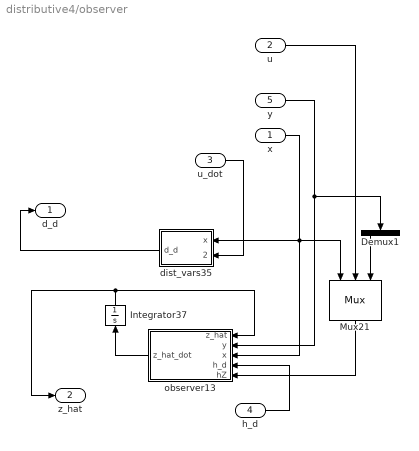
== system distributive4/observer ==
  x : Inport
  u : Inport  Port=2
  u_dot : Inport  Port=3
  h_d : Inport  Port=4
  y : Inport  Port=5
  Demux1 : Demux  Outputs=2
  Integrator37 : Integrator  InitialCondition=[0;0]
  Mux21 : Mux  Inputs=3
      settings: DisplayOption=signals
  dist_vars35 : Subsystem
      settings: PortSchema="{\"entries\":[{\"content\":{\"sides\":[{\"content\":{\"connectorIds\":[\"Out1\"]},\"type\":\"ConnectorPlacement.EquallySpacedRectSide\",\"uuid\":\"c6804a03-85ed-4e19-a8b2-23b3b91cc999\"},{\"content\":{\"connectorIds\":[\"In1\",\"In2\"],\"side\":\"RIGHT\"},\"type\":\"ConnectorPlacement.EquallySpacedRectSide\",\"uuid\":\"3893e005-dabd-44b9-aa2f-690b9b6a2b6d\"},{\"content\":{\"connectorIds\":[],\"side\":\"TOP\"},\"type\":\"ConnectorPlacement.EquallySpacedRectSide\",\"uuid\":\"9986ad97-c002-4a16-bb79-a95333cc5799\"}]},\"type\":\"ConnectorPlacement.EquallySpacedConnector\",\"uuid\":\"d796f436-4cc2-4114-998c-ef0d57f68d4d\"}],\"packageUris\":[\"http://schema.mathworks.com/mf0/Connector/R2020b\"],\"version\":\"1.0\"}"
  observer13 : MATLAB Function  TreatAsAtomicUnit=on
  d_d : Outport
  z_hat : Outport  Port=2
  wires:
  Integrator37/1 -> z_hat/1, observer13/1(z_hat)
  x/1 -> observer13/3(x), Mux21/1, dist_vars35/1(x)
  dist_vars35/1(d_d) -> d_d/1
  Mux21/1 -> observer13/5(hZ)
  observer13/1(z_hat_dot) -> Integrator37/1
  y/1 -> Demux1/1, observer13/2(y)
  u_dot/1 -> dist_vars35/2(u_dot)
  h_d/1 -> observer13/4(h_d)
  u/1 -> Mux21/2
  Demux1/1 -> Mux21/3

== system distributive4/observer2 ==
  x : Inport
  u : Inport  Port=2
  u_dot : Inport  Port=3
  h_d : Inport  Port=4
  y : Inport  Port=5
  Demux1 : Demux  Outputs=2
  Integrator37 : Integrator  InitialCondition=[0;0]
  Mux21 : Mux  Inputs=3
      settings: DisplayOption=signals
  dist_vars35 : Subsystem
      settings: PortSchema="{\"entries\":[{\"content\":{\"sides\":[{\"content\":{\"connectorIds\":[\"Out1\"]},\"type\":\"ConnectorPlacement.EquallySpacedRectSide\",\"uuid\":\"c6804a03-85ed-4e19-a8b2-23b3b91cc999\"},{\"content\":{\"connectorIds\":[\"In1\",\"In2\"],\"side\":\"RIGHT\"},\"type\":\"ConnectorPlacement.EquallySpacedRectSide\",\"uuid\":\"3893e005-dabd-44b9-aa2f-690b9b6a2b6d\"},{\"content\":{\"connectorIds\":[],\"side\":\"TOP\"},\"type\":\"ConnectorPlacement.EquallySpacedRectSide\",\"uuid\":\"9986ad97-c002-4a16-bb79-a95333cc5799\"}]},\"type\":\"ConnectorPlacement.EquallySpacedConnector\",\"uuid\":\"d796f436-4cc2-4114-998c-ef0d57f68d4d\"}],\"packageUris\":[\"http://schema.mathworks.com/mf0/Connector/R2020b\"],\"version\":\"1.0\"}"
  observer13 : MATLAB Function  TreatAsAtomicUnit=on
  d_d : Outport
  z_hat : Outport  Port=2
  wires:
  Integrator37/1 -> z_hat/1, observer13/1(z_hat)
  x/1 -> observer13/3(x), Mux21/1, dist_vars35/1(x)
  dist_vars35/1(d_d) -> d_d/1
  Mux21/1 -> observer13/5(hZ)
  observer13/1(z_hat_dot) -> Integrator37/1
  y/1 -> Demux1/1, observer13/2(y)
  u_dot/1 -> dist_vars35/2(u_dot)
  h_d/1 -> observer13/4(h_d)
  u/1 -> Mux21/2
  Demux1/1 -> Mux21/3

== system distributive4/observer3 ==
  x : Inport
  u : Inport  Port=2
  u_dot : Inport  Port=3
  h_d : Inport  Port=4
  y : Inport  Port=5
  Demux1 : Demux  Outputs=2
  Integrator37 : Integrator  InitialCondition=[0;0]
  Mux21 : Mux  Inputs=3
      settings: DisplayOption=signals
  dist_vars35 : Subsystem
      settings: PortSchema="{\"entries\":[{\"content\":{\"sides\":[{\"content\":{\"connectorIds\":[\"Out1\"]},\"type\":\"ConnectorPlacement.EquallySpacedRectSide\",\"uuid\":\"c6804a03-85ed-4e19-a8b2-23b3b91cc999\"},{\"content\":{\"connectorIds\":[\"In1\",\"In2\"],\"side\":\"RIGHT\"},\"type\":\"ConnectorPlacement.EquallySpacedRectSide\",\"uuid\":\"3893e005-dabd-44b9-aa2f-690b9b6a2b6d\"},{\"content\":{\"connectorIds\":[],\"side\":\"TOP\"},\"type\":\"ConnectorPlacement.EquallySpacedRectSide\",\"uuid\":\"9986ad97-c002-4a16-bb79-a95333cc5799\"}]},\"type\":\"ConnectorPlacement.EquallySpacedConnector\",\"uuid\":\"d796f436-4cc2-4114-998c-ef0d57f68d4d\"}],\"packageUris\":[\"http://schema.mathworks.com/mf0/Connector/R2020b\"],\"version\":\"1.0\"}"
  observer13 : MATLAB Function  TreatAsAtomicUnit=on
  d_d : Outport
  z_hat : Outport  Port=2
  wires:
  Integrator37/1 -> z_hat/1, observer13/1(z_hat)
  x/1 -> observer13/3(x), Mux21/1, dist_vars35/1(x)
  dist_vars35/1(d_d) -> d_d/1
  Mux21/1 -> observer13/5(hZ)
  observer13/1(z_hat_dot) -> Integrator37/1
  y/1 -> Demux1/1, observer13/2(y)
  u_dot/1 -> dist_vars35/2(u_dot)
  h_d/1 -> observer13/4(h_d)
  u/1 -> Mux21/2
  Demux1/1 -> Mux21/3

== system distributive4/Subsystem/dist_vars32 ==
  note: h_d1
  x : Inport
  u : Inport  Port=2
  t : Inport  Port=3
  Derivative1 : Derivative
  Integrator1 : Integrator
  MATLAB Function : MATLAB Function  TreatAsAtomicUnit=on
  MATLAB Function5 : MATLAB Function  TreatAsAtomicUnit=on
  h_d : Outport
  h : Outport  Port=2
  d_d : Outport  Port=3
  wires:
  Integrator1/1 -> h/1, MATLAB Function5/2(h)
  MATLAB Function5/1(h_dot) -> Integrator1/1
  x/1 -> MATLAB Function5/3(x), MATLAB Function/1(x)
  MATLAB Function/1(d_d) -> d_d/1
  MATLAB Function5/2(h_d) -> h_d/1
  u/1 -> Derivative1/1
  Derivative1/1 -> MATLAB Function5/1(u_dot)
  t/1 -> MATLAB Function5/4(t)

== system distributive4/Subsystem1/measurements ==
  u : Inport
  Derivative2 : Derivative
  IC : InitialCondition  Value=0
  Integrator1 : Integrator
  MATLAB Function1 : MATLAB Function  TreatAsAtomicUnit=on
  MATLAB Function5 : MATLAB Function  TreatAsAtomicUnit=on
  y_L : Outport
  h : Outport  Port=2
  wires:
  Integrator1/1 -> IC/1
  MATLAB Function5/1(h_dot) -> Integrator1/1
  u/1 -> MATLAB Function1/2(u), Derivative2/1
  MATLAB Function1/1(y_L) -> y_L/1
  Derivative2/1 -> MATLAB Function5/1(u_dot)
  IC/1 -> MATLAB Function5/2(h), MATLAB Function1/1(h), h/1

== system distributive4/Subsystem10/dist_vars1 ==
  x : Inport
  u_dot : Inport  Port=2
  t : Inport  Port=3
  Integrator2 : Integrator
  MATLAB Function : MATLAB Function  TreatAsAtomicUnit=on
  MATLAB Function5 : MATLAB Function  TreatAsAtomicUnit=on
  h_d : Outport
  h : Outport  Port=2
  d_d : Outport  Port=3
  wires:
  x/1 -> MATLAB Function5/3(x), MATLAB Function/1(x)
  MATLAB Function/1(d_d) -> d_d/1
  u_dot/1 -> MATLAB Function5/1(u_dot)
  MATLAB Function5/2(h_d) -> h_d/1
  MATLAB Function5/1(h_dot) -> Integrator2/1
  t/1 -> MATLAB Function5/4(t)
  Integrator2/1 -> MATLAB Function5/2(h), h/1

== system distributive4/Subsystem12/dist_vars15 ==
  u_dot : Inport
  x : Inport  Port=2
  Integrator2 : Integrator
  Integrator3 : Integrator
  MATLAB Function : MATLAB Function  TreatAsAtomicUnit=on
  MATLAB Function1 : MATLAB Function  TreatAsAtomicUnit=on
  h_d_dot : Outport
  d_d : Outport  Port=2
  h_d : Outport  Port=3
  wires:
  MATLAB Function/1(d_d) -> d_d/1
  MATLAB Function1/1(h_dot) -> Integrator3/1
  u_dot/1 -> MATLAB Function1/1(u_dot)
  MATLAB Function1/2(h_d_dot) -> h_d_dot/1, Integrator2/1
  x/1 -> MATLAB Function1/3(x), MATLAB Function/1(x)
  Integrator3/1 -> MATLAB Function1/2(h)
  Integrator2/1 -> h_d/1

== system distributive4/Subsystem13/dist_vars1 ==
  x : Inport
  u_dot : Inport  Port=2
  t : Inport  Port=3
  Integrator2 : Integrator
  MATLAB Function : MATLAB Function  TreatAsAtomicUnit=on
  MATLAB Function5 : MATLAB Function  TreatAsAtomicUnit=on
  h_d : Outport
  h : Outport  Port=2
  d_d : Outport  Port=3
  wires:
  x/1 -> MATLAB Function5/3(x), MATLAB Function/1(x)
  MATLAB Function/1(d_d) -> d_d/1
  u_dot/1 -> MATLAB Function5/1(u_dot)
  MATLAB Function5/2(h_d) -> h_d/1
  MATLAB Function5/1(h_dot) -> Integrator2/1
  t/1 -> MATLAB Function5/4(t)
  Integrator2/1 -> MATLAB Function5/2(h), h/1

== system distributive4/Subsystem15/dist_vars15 ==
  u_dot : Inport
  x : Inport  Port=2
  Integrator2 : Integrator
  Integrator3 : Integrator
  MATLAB Function : MATLAB Function  TreatAsAtomicUnit=on
  MATLAB Function1 : MATLAB Function  TreatAsAtomicUnit=on
  h_d_dot : Outport
  d_d : Outport  Port=2
  h_d : Outport  Port=3
  wires:
  MATLAB Function/1(d_d) -> d_d/1
  MATLAB Function1/1(h_dot) -> Integrator3/1
  u_dot/1 -> MATLAB Function1/1(u_dot)
  MATLAB Function1/2(h_d_dot) -> h_d_dot/1, Integrator2/1
  x/1 -> MATLAB Function1/3(x), MATLAB Function/1(x)
  Integrator3/1 -> MATLAB Function1/2(h)
  Integrator2/1 -> h_d/1

== system distributive4/Subsystem16/dist_vars14 ==
  x : Inport
  u_dot : Inport  Port=2
  t : Inport  Port=3
  Integrator2 : Integrator
  MATLAB Function : MATLAB Function  TreatAsAtomicUnit=on
  MATLAB Function5 : MATLAB Function  TreatAsAtomicUnit=on
  h : Outport
  h_d : Outport  Port=2
  d_d : Outport  Port=3
  wires:
  x/1 -> MATLAB Function5/3(x), MATLAB Function/1(x)
  MATLAB Function/1(d_d) -> d_d/1
  u_dot/1 -> MATLAB Function5/1(u_dot)
  MATLAB Function5/2(h_d) -> h_d/1
  MATLAB Function5/1(h_dot) -> Integrator2/1
  t/1 -> MATLAB Function5/4(t)
  Integrator2/1 -> h/1, MATLAB Function5/2(h)

== system distributive4/Subsystem2/Subsystem4 ==
  x : Inport
  u : Inport  Port=2
  Derivative1 : Derivative
  Integrator2 : Integrator
  estimator : MATLAB Function  TreatAsAtomicUnit=on
  measurements : Subsystem
      settings: PortSchema="{\"entries\":[{\"content\":{\"sides\":[{\"content\":{\"connectorIds\":[]},\"type\":\"ConnectorPlacement.EquallySpacedRectSide\",\"uuid\":\"c6804a03-85ed-4e19-a8b2-23b3b91cc999\"},{\"content\":{\"connectorIds\":[\"Out1\",\"In1\",\"Out2\"],\"side\":\"RIGHT\"},\"type\":\"ConnectorPlacement.EquallySpacedRectSide\",\"uuid\":\"3893e005-dabd-44b9-aa2f-690b9b6a2b6d\"},{\"content\":{\"connectorIds\":[],\"side\":\"TOP\"},\"type\":\"ConnectorPlacement.EquallySpacedRectSide\",\"uuid\":\"9986ad97-c002-4a16-bb79-a95333cc5799\"}]},\"type\":\"ConnectorPlacement.EquallySpacedConnector\",\"uuid\":\"d796f436-4cc2-4114-998c-ef0d57f68d4d\"}],\"packageUris\":[\"http://schema.mathworks.com/mf0/Connector/R2020b\"],\"version\":\"1.0\"}"
  d_d_hat : Outport
  y_d_hat : Outport  Port=2
  h_d_hat : Outport  Port=3
  u_dot : Outport  Port=4
  wires:
  estimator/1(y_d_hat) -> y_d_hat/1
  estimator/4(d_d_hat) -> d_d_hat/1
  u/1 -> estimator/2(u), Derivative1/1
  Integrator2/1 -> estimator/1(h)
  Derivative1/1 -> u_dot/1, estimator/3(u_dot)
  x/1 -> estimator/4(x)
  estimator/2(h_dot) -> Integrator2/1
  estimator/3(h_d_hat) -> h_d_hat/1

== system distributive4/Subsystem3/dist_vars14 ==
  x : Inport
  u_dot : Inport  Port=2
  t : Inport  Port=3
  Integrator2 : Integrator
  MATLAB Function : MATLAB Function  TreatAsAtomicUnit=on
  MATLAB Function5 : MATLAB Function  TreatAsAtomicUnit=on
  h : Outport
  h_d : Outport  Port=2
  d_d : Outport  Port=3
  wires:
  x/1 -> MATLAB Function5/3(x), MATLAB Function/1(x)
  MATLAB Function/1(d_d) -> d_d/1
  u_dot/1 -> MATLAB Function5/1(u_dot)
  MATLAB Function5/2(h_d) -> h_d/1
  MATLAB Function5/1(h_dot) -> Integrator2/1
  t/1 -> MATLAB Function5/4(t)
  Integrator2/1 -> h/1, MATLAB Function5/2(h)

== system distributive4/Subsystem5/dist_vars1 ==
  x : Inport
  u_dot : Inport  Port=2
  t : Inport  Port=3
  Integrator2 : Integrator
  MATLAB Function : MATLAB Function  TreatAsAtomicUnit=on
  MATLAB Function5 : MATLAB Function  TreatAsAtomicUnit=on
  h_d : Outport
  h : Outport  Port=2
  d_d : Outport  Port=3
  wires:
  x/1 -> MATLAB Function5/3(x), MATLAB Function/1(x)
  MATLAB Function/1(d_d) -> d_d/1
  u_dot/1 -> MATLAB Function5/1(u_dot)
  MATLAB Function5/2(h_d) -> h_d/1
  MATLAB Function5/1(h_dot) -> Integrator2/1
  t/1 -> MATLAB Function5/4(t)
  Integrator2/1 -> MATLAB Function5/2(h), h/1

== system distributive4/Subsystem7/dist_vars15 ==
  u_dot : Inport
  x : Inport  Port=2
  Integrator2 : Integrator
  Integrator3 : Integrator
  MATLAB Function : MATLAB Function  TreatAsAtomicUnit=on
  MATLAB Function1 : MATLAB Function  TreatAsAtomicUnit=on
  h_d_dot : Outport
  d_d : Outport  Port=2
  h_d : Outport  Port=3
  wires:
  MATLAB Function/1(d_d) -> d_d/1
  MATLAB Function1/1(h_dot) -> Integrator3/1
  u_dot/1 -> MATLAB Function1/1(u_dot)
  MATLAB Function1/2(h_d_dot) -> h_d_dot/1, Integrator2/1
  x/1 -> MATLAB Function1/3(x), MATLAB Function/1(x)
  Integrator3/1 -> MATLAB Function1/2(h)
  Integrator2/1 -> h_d/1

== system distributive4/Subsystem8/dist_vars14 ==
  x : Inport
  u_dot : Inport  Port=2
  t : Inport  Port=3
  Integrator2 : Integrator
  MATLAB Function : MATLAB Function  TreatAsAtomicUnit=on
  MATLAB Function5 : MATLAB Function  TreatAsAtomicUnit=on
  h : Outport
  h_d : Outport  Port=2
  d_d : Outport  Port=3
  wires:
  x/1 -> MATLAB Function5/3(x), MATLAB Function/1(x)
  MATLAB Function/1(d_d) -> d_d/1
  u_dot/1 -> MATLAB Function5/1(u_dot)
  MATLAB Function5/2(h_d) -> h_d/1
  MATLAB Function5/1(h_dot) -> Integrator2/1
  t/1 -> MATLAB Function5/4(t)
  Integrator2/1 -> h/1, MATLAB Function5/2(h)

== system distributive4/observer/dist_vars35 ==
  x : Inport
  u_dot : Inport  Port=2
  Integrator1 : Integrator
  MATLAB Function : MATLAB Function  TreatAsAtomicUnit=on
  MATLAB Function5 : MATLAB Function  TreatAsAtomicUnit=on
  d_d : Outport
  wires:
  Integrator1/1 -> MATLAB Function5/2(h)
  MATLAB Function5/1(h_dot) -> Integrator1/1
  u_dot/1 -> MATLAB Function5/1(u_dot)
  MATLAB Function/1(d_d) -> d_d/1
  x/1 -> MATLAB Function5/3(x), MATLAB Function/1(x)

== system distributive4/observer2/dist_vars35 ==
  x : Inport
  u_dot : Inport  Port=2
  Integrator1 : Integrator
  MATLAB Function : MATLAB Function  TreatAsAtomicUnit=on
  MATLAB Function5 : MATLAB Function  TreatAsAtomicUnit=on
  d_d : Outport
  wires:
  Integrator1/1 -> MATLAB Function5/2(h)
  MATLAB Function5/1(h_dot) -> Integrator1/1
  u_dot/1 -> MATLAB Function5/1(u_dot)
  MATLAB Function/1(d_d) -> d_d/1
  x/1 -> MATLAB Function5/3(x), MATLAB Function/1(x)

== system distributive4/observer3/dist_vars35 ==
  x : Inport
  u_dot : Inport  Port=2
  Integrator1 : Integrator
  MATLAB Function : MATLAB Function  TreatAsAtomicUnit=on
  MATLAB Function5 : MATLAB Function  TreatAsAtomicUnit=on
  d_d : Outport
  wires:
  Integrator1/1 -> MATLAB Function5/2(h)
  MATLAB Function5/1(h_dot) -> Integrator1/1
  u_dot/1 -> MATLAB Function5/1(u_dot)
  MATLAB Function/1(d_d) -> d_d/1
  x/1 -> MATLAB Function5/3(x), MATLAB Function/1(x)

== system distributive4/Subsystem2/Subsystem4/measurements ==
  u : Inport
  Derivative2 : Derivative
  IC : InitialCondition  Value=0
  Integrator1 : Integrator
  MATLAB Function1 : MATLAB Function  TreatAsAtomicUnit=on
  MATLAB Function5 : MATLAB Function  TreatAsAtomicUnit=on
  y_L : Outport
  h : Outport  Port=2
  wires:
  Integrator1/1 -> IC/1
  MATLAB Function5/1(h_dot) -> Integrator1/1
  u/1 -> MATLAB Function1/2(u), Derivative2/1
  MATLAB Function1/1(y_L) -> y_L/1
  Derivative2/1 -> MATLAB Function5/1(u_dot)
  IC/1 -> MATLAB Function5/2(h), MATLAB Function1/1(h), h/1

== matlab function distributive4/Subsystem7/observer5 ==
  data: z_hat input; y input; x input; h_d input; u input; A parameter; B parameter; z_hat_dot output; C_bar parameter; S parameter; Gamma parameter; h_d_dot input size=1; d_d input; L parameter; G parameter
function z_hat_dot   = fcn(z_hat,y,x,h_d,u,A, B, C_bar,S,Gamma,h_d_dot,d_d,L,G)
y_L=y(1); % Y=y_L
y_d=y_L*(x/L)^2;
y_hat = z_hat(1);

z=[y_d;h_d];
f_hat = h_d_dot;
g_hat = [A*y_hat + B*d_d*u;
            f_hat         ];
% z_hat_dot = Gamma*z_hat + g_hat - (S\C_bar')*(y_hat-y);  y = Cz



% function z_hat_dot   = fcn(z_hat,y,x,h_d,C_bar,S,Gamma,hZ,V,W, L)
% %y_hat=z_hat(1);
%  y_L=y(1); % Y=y_L
%  y_d=y_L*(x/L)^2;
% z=[y_d;h_d];
                                                   % hg = (2x1) = (2x8)*(8x1)
% G= S\C_bar;
% 
% z_hat_dot = Gamma*z_hat + g_hat + G*C_bar'*(z-z_hat); %G*C_bar*(z-z_hat); %
z_hat_dot = Gamma*z_hat + g_hat + G*C_bar*(z-z_hat); %
% end


% z_hat_dot = Gamma*z_hat + g_hat - (S\C_bar')*(y_hat-y);

== matlab function distributive4/Subsystem10/dist_vars1/MATLAB Function5 ==
  data: h_dot output; h_d output; u_dot input; h input; x input; alpha parameter; gamma parameter; beta parameter; L parameter; t input
function [h_dot,h_d]  = fcn(u_dot,h,x,alpha, gamma, beta,L,t)

delta_h=25*t;
h_dot = alpha*u_dot - beta*abs(u_dot)*h - gamma*u_dot*abs(h)+delta_h;
%h_d_dot = h_dot*(x/L)^2;
h_d=h*(x/L)^2;

== matlab function distributive4/Subsystem4/u_ref_dot6 ==
  data: h_d_ref input; z_hat input; u_ref_dot output size=1; alpha parameter size=1; k1 parameter size=1; k2 parameter size=1; x input; L parameter; h_d_dot input
function u_ref_dot = fcn(h_d_ref,z_hat,alpha,k1,k2,x,L,h_d_dot)
h_d_hat=z_hat(2);
% syms c1 c2 k1 k2 alfa betta rho sigma

e_h = h_d_hat - h_d_ref;
alpha_d = alpha*(x/L)^2;

%u_dot =  k1*sign(e) + k2*e; %con este "x" converge mejor ; ver porque debe tener signos [+]
%u_ref_dot= k1*sign(e) + k2*e; %este es el ùnico que sí controla el modelo de micky con A_h=0.9e-6

%u_dot =  (1/A_h)*(-k1*sign(e)*sqrt(abs(e)) - k2*e ); %este tambien

%u_ref_dot=(1/alpha_d)*(-k1*sign(e)*sqrt(abs(e)) - k2*e);
u_ref_dot=(1/alpha_d)*( k1*sign(e_h)*sqrt(abs(e_h)) + k2*e_h );

%u_dot =  (1/A_h)*(- k1*sign(e) - k2*e + hd_dot); % este es el bueno
%u_ref_dot=(1/alpha_d)*(-k1*sign(e) - k2*e + h_d_dot);

== matlab function distributive4/Subsystem3/v6 ==
  data: d_d input; v output; u input; h_d input; h input; d_p parameter
% function v = fcn(d_d,u,h_d)
% 
% v=d_d*u-h_d;

function v = fcn(d_d,u,h_d,h, d_p)

%v=d_d*u-h_d;
v=[ d_p*u-h ; d_d*u-h_d ];

== matlab function distributive4/Subsystem3/y8 ==
  data: y output; v input; Y input; Y_dot output; A parameter; B parameter; C parameter; t input
function [y,Y_dot] = fcn(v,Y, A, B, C,t)

delta_y = [30;0];
Y_dot = A*Y + B*v + delta_y;
y=C*Y;

== matlab function distributive4/dist_vars22/MATLAB Function ==
  data: x input; L parameter; d_p parameter; d_d output
function d_d   = fcn(x,L, d_p)

d_d = (x/L)*(x/L)*d_p;

== matlab function distributive4/dist_vars22/MATLAB Function5 ==
  data: u_dot input; h_dot output; h input; x input; alpha parameter; gamma parameter; beta parameter; L parameter; h_d output; h_d_dot output
function [h_dot,h_d,h_d_dot] = fcn(u_dot,h,x,alpha, gamma, beta,L)


h_dot = alpha*u_dot - beta*abs(u_dot)*h - gamma*u_dot*abs(h);
h_d=h*(x/L)^2;
h_d_dot=h_dot*(x/L)^2;

== matlab function distributive4/dist_vars23/MATLAB Function ==
  data: x input; L parameter; d_p parameter; d_d output
function d_d   = fcn(x,L, d_p)

d_d = (x/L)*(x/L)*d_p;

== matlab function distributive4/dist_vars23/MATLAB Function5 ==
  data: u_dot input; h_dot output; h input; x input; alpha parameter; gamma parameter; beta parameter; L parameter; h_d output; h_d_dot output
function [h_dot,h_d,h_d_dot] = fcn(u_dot,h,x,alpha, gamma, beta,L)


h_dot = alpha*u_dot - beta*abs(u_dot)*h - gamma*u_dot*abs(h);
h_d=h*(x/L)^2;
h_d_dot=h_dot*(x/L)^2;

== matlab function distributive4/dist_vars24/MATLAB Function ==
  data: x input; L parameter; d_p parameter; d_d output
function d_d   = fcn(x,L, d_p)

d_d = (x/L)*(x/L)*d_p;

== matlab function distributive4/dist_vars24/MATLAB Function5 ==
  data: u_dot input; h_dot output; h input; x input; alpha parameter; gamma parameter; beta parameter; L parameter; h_d output; h_d_dot output
function [h_dot,h_d,h_d_dot] = fcn(u_dot,h,x,alpha, gamma, beta,L)


h_dot = alpha*u_dot - beta*abs(u_dot)*h - gamma*u_dot*abs(h);
h_d=h*(x/L)^2;
h_d_dot = h_dot*(x/L)^2;

== matlab function distributive4/dist_vars25/MATLAB Function ==
  data: x input; L parameter; d_p parameter; d_d output
function d_d   = fcn(x,L, d_p)

d_d = (x/L)*(x/L)*d_p;

== matlab function distributive4/dist_vars25/MATLAB Function5 ==
  data: u_dot input; h_dot output; h input; x input; alpha parameter; gamma parameter; beta parameter; L parameter; h_d output; h_d_dot output
function [h_dot,h_d,h_d_dot] = fcn(u_dot,h,x,alpha, gamma, beta,L)


h_dot = alpha*u_dot - beta*abs(u_dot)*h - gamma*u_dot*abs(h);
h_d=h*(x/L)^2;
h_d_dot = h_dot*(x/L)^2;

== matlab function distributive4/errors11 ==
  data: z_hat input; y input; h_d input; e_y output; e_h output; e_y2 output; e_h2 output; y_ref input; h_d_ref input
function [e_y,e_h,e_y2,e_h2]   = fcn(z_hat,y,h_d,y_ref, h_d_ref)
e_y=z_hat(1)-y;
e_h=z_hat(2)-h_d;
e_y2=y_ref-y;
e_h2=h_d_ref-h_d;

== matlab function distributive4/Subsystem10/v3 ==
  data: d_d input; v output; u input; h_d input; h input; d_p parameter
% function v = fcn(d_d,u,h_d)
% 
% v=d_d*u-h_d;

function v = fcn(d_d,u,h_d,h, d_p)

%v=d_d*u-h_d;
v=[ d_p*u-h ; d_d*u-h_d ];

== matlab function distributive4/errors12 ==
  data: z_hat input; y input; h_d input; e_y output; e_h output; e_y2 output; e_h2 output; y_ref input; h_d_ref input
function [e_y,e_h,e_y2,e_h2]   = fcn(z_hat,y,h_d,y_ref, h_d_ref)
e_y=z_hat(1)-y;
e_h=z_hat(2)-h_d;
e_y2=y_ref-y;
e_h2=h_d_ref-h_d;

== matlab function distributive4/h_d_ref10 ==
  data: u input; Y_ref input; Y_ref_dot input; Y input; h_d_ref output; A parameter; B parameter; kappa1 parameter; d_d input
function h_d_ref = fcn(u,Y_ref, Y_ref_dot,Y, A, B, kappa1, d_d)


Y_tilde=Y-Y_ref;
h_d_ref=B\((A + kappa1)*Y_tilde + A*Y_ref -Y_ref_dot +B*d_d*u);

== matlab function distributive4/h_d_ref11 ==
  data: u input; Y_ref input; Y_ref_dot input; Y input; h_d_ref output; A parameter; B parameter; kappa1 parameter; d_d input
function h_d_ref = fcn(u,Y_ref, Y_ref_dot,Y, A, B, kappa1, d_d)


Y_tilde=Y-Y_ref;
h_d_ref=B\((A + kappa1)*Y_tilde + A*Y_ref -Y_ref_dot +B*d_d*u);
